simulink subsystem "rocket_flight"  (R2024b)
settings: Solver=VariableStepAuto  StartTime=0.0  StopTime=10.0  RelTol=1e-3
undefined symbols (not defined in the file or in its folder): location, Mdot, OR_cg, rail_angle_pitch, rail_angle_roll, rail_angle_yaw, sim_time, time_idle
libraries: shared6dof x1
settings Model: Creator=joedo  LastModifiedBy=finnb

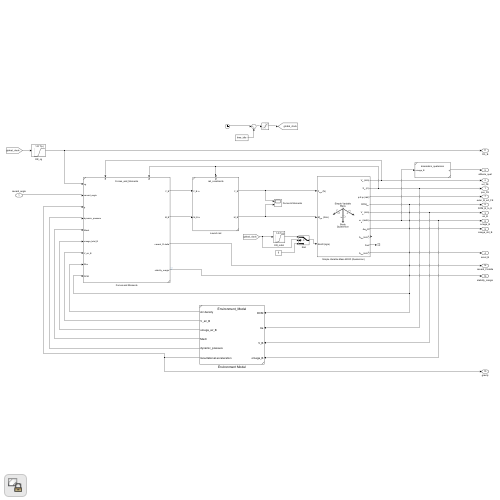
[thumbnail: Simulink's stored preview of the top-level diagram]
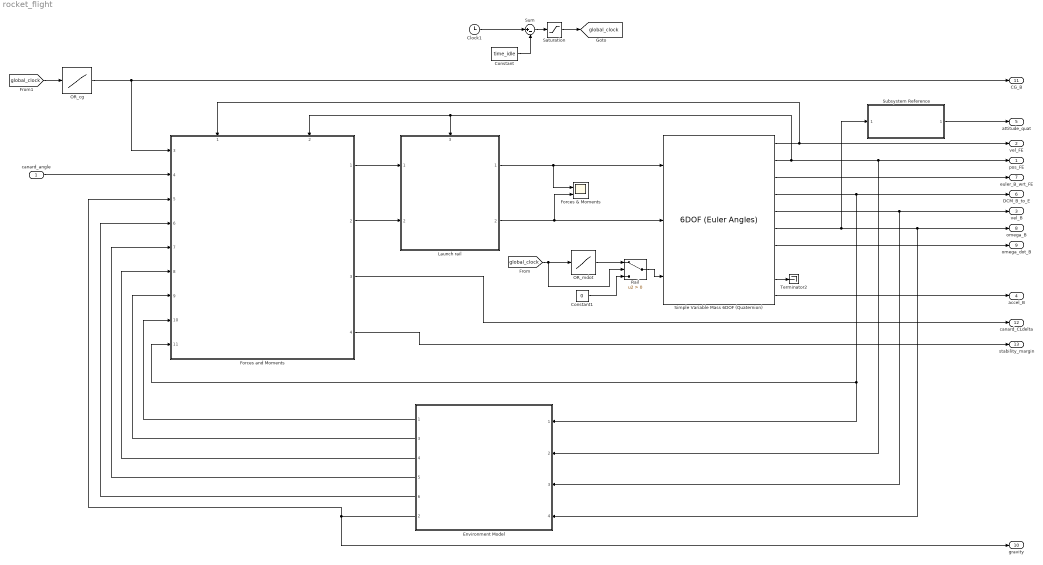
== system rocket_flight ==
  canard_angle : Inport
  Clock1 : Clock
  Constant : Constant  Value=time_idle
  Constant1 : Constant  Value=0
  Environment Model : Subsystem  ReferencedSubsystem=Environment_Model
      settings: PortSchema="{\"entries\":[{\"content\":{\"sides\":[{\"content\":{\"connectorIds\":[\"In1\",\"In2\",\"In3\",\"In4\"]},\"type\":\"ConnectorPlacement.EquallySpacedRectSide\",\"uuid\":\"2a81b9c5-b150-4b95-94af-394a03d0678a\"},{\"content\":{\"connectorIds\":[\"Out1\",\"Out3\",\"Out4\",\"Out5\",\"Out6\",\"Out2\"],\"side\":\"RIGHT\"},\"type\":\"ConnectorPlacement.EquallySpacedRectSide\",\"uuid\":\"876dc6e2-e5c6-4258-adc0-40f09f61a15a\"},{\"content\":{\"side\":\"TOP\"},\"type\":\"ConnectorPlacement.EquallySpacedRectSide\",\"uuid\":\"30ca8b3b-9b10-4b0a-a581-f2563a0e4844\"}]},\"type\":\"ConnectorPlacement.EquallySpacedConnector\",\"uuid\":\"0a44bd71-bf6b-4260-a474-a2581db635e7\"}],\"packageUris\":[\"http://schema.mathworks.com/mf0/Connector/R2020b\"],\"version\":\"1.0\"}"
  Forces & Moments : Scope  NumInputPorts=2
  "Forces and Moments " : Subsystem  ReferencedSubsystem=Forces_and_Moments
      settings: PortSchema="{\"entries\":[{\"content\":{\"sides\":[{\"content\":{\"connectorIds\":[\"In3\",\"In4\",\"In5\",\"In6\",\"In7\",\"In8\",\"In9\",\"In10\",\"In11\"]},\"type\":\"ConnectorPlacement.EquallySpacedRectSide\",\"uuid\":\"2d9b15f2-fc7e-4399-b4ca-f7faa58838df\"},{\"content\":{\"connectorIds\":[\"Out1\",\"Out2\",\"Out3\",\"Out4\"],\"side\":\"RIGHT\"},\"type\":\"ConnectorPlacement.EquallySpacedRectSide\",\"uuid\":\"cd9b89d4-ce85-488b-9a3f-64297ccf9b96\"},{\"content\":{\"connectorIds\":[\"In1\",\"In2\"],\"side\":\"TOP\"},\"type\":\"ConnectorPlacement.EquallySpacedRectSide\",\"uuid\":\"472a10a7-0072-45c6-a8aa-5eaf234894da\"}]},\"type\":\"ConnectorPlacement.EquallySpacedConnector\",\"uuid\":\"79d150c0-9861-42cf-8cdc-8f9e609deb28\"}],\"packageUris\":[\"http://schema.mathworks.com/mf0/Connector/R2020b\"],\"version\":\"1.0\"}"
  Launch rail : Subsystem  ReferencedSubsystem=rail_constraints
      settings: PortSchema="{\"entries\":[{\"content\":{\"sides\":[{\"content\":{\"connectorIds\":[\"In1\",\"In2\"]},\"type\":\"ConnectorPlacement.EquallySpacedRectSide\",\"uuid\":\"f8bc89cf-4366-4095-a699-e573bc22001a\"},{\"content\":{\"connectorIds\":[\"Out1\",\"Out2\"],\"side\":\"RIGHT\"},\"type\":\"ConnectorPlacement.EquallySpacedRectSide\",\"uuid\":\"f55d6fa0-3d5e-48fa-b07b-9e72276225fb\"},{\"content\":{\"connectorIds\":[\"In3\"],\"side\":\"TOP\"},\"type\":\"ConnectorPlacement.EquallySpacedRectSide\",\"uuid\":\"5696589c-23a4-46a9-b349-1864b914459a\"}]},\"type\":\"ConnectorPlacement.EquallySpacedConnector\",\"uuid\":\"1b8f695c-cf97-4880-abd1-8dadf97d6ecb\"}],\"packageUris\":[\"http://schema.mathworks.com/mf0/Connector/R2020b\"],\"version\":\"1.0\"}"
  OR_cg : Lookup_n-D  NumberOfTableDimensions=1  BreakpointsForDimension1=sim_time  Table=OR_cg  InternalRulePriority=Speed  RndMeth=Simplest
  OR_mdot : Lookup_n-D  NumberOfTableDimensions=1  BreakpointsForDimension1=sim_time  Table=Mdot  InternalRulePriority=Speed  RndMeth=Simplest
  Rail : Switch  Criteria=u2 > Threshold  SaturateOnIntegerOverflow=off  InputSameDT=off
  Saturation : Saturate  UpperLimit=inf  LowerLimit=0
  Simple Variable Mass 6DOF (Quaternion) : shared6dof/6DOF (Euler Angles)  units=Metric (MKS)  mtype=Simple Variable  rep=Quaternion  xme_0=[location(1) 0 0]  Vm_0=[0 0 0]  eul_0=[rail_angle_roll, rail_angle_pitch, rail_angle_yaw]  pm_0=[0 0 0]  mass_0=total_mass_0  mass_e=total_mass_d  mass_f=total_mass_0  inertia=eye(3)  inertia_e=I_d  inertia_f=I_0  k_quat=1.0  vre_flag=off  abi_flag=on  aMode=0  xme_statename=''  Vm_statename=''  eul_statename=''  quat_statename=''  pm_statename=''  mass_statename=''
      settings: LibrarySourceBlock=aerolib6dof2/Simple Variable Mass 6DOF (Quaternion)
  Subsystem Reference : Subsystem  ReferencedSubsystem=kinematics_quaternion
  Sum : Sum  Inputs=|+-
  Terminator2 : Terminator
  pos_FE : Outport
  vel_FE : Outport  Port=2
  vel_B : Outport  Port=3  PortDimensions=3
  accel_B : Outport  Port=4  PortDimensions=3
  attitude_quat : Outport  Port=5
  DCM_B_to_E : Outport  Port=6
  euler_B_wrt_FE : Outport  Port=7
  omega_B : Outport  Port=8
  omega_dot_B : Outport  Port=9
  gravity : Outport  Port=10
  CG_B : Outport  Port=11
  canard_CLdelta : Outport  Port=12
  stability_margin : Outport  Port=13
  tag scope: global_clock=global
  wires:
  "Forces and Moments "/4 -> stability_margin/1
  "Forces and Moments "/3 -> canard_CLdelta/1
  "Forces and Moments "/2 -> Launch rail/2
  "Forces and Moments "/1 -> Launch rail/1
  Environment Model/6 -> "Forces and Moments "/6
  Environment Model/3 -> "Forces and Moments "/9
  Subsystem Reference/1 -> attitude_quat/1
  Saturation/1 -> [global_clock]
  Constant/1 -> Sum/2
  Sum/1 -> Saturation/1
  Clock1/1 -> Sum/1
  OR_cg/1 -> "Forces and Moments "/3, CG_B/1
  [global_clock] -> OR_cg/1
  Constant1/1 -> Rail/3
  Rail/1 -> Simple Variable Mass 6DOF (Quaternion)/3
  [global_clock] -> OR_mdot/1, Rail/2
  Simple Variable Mass 6DOF (Quaternion)/4 -> Environment Model/1, "Forces and Moments "/11, DCM_B_to_E/1
  Simple Variable Mass 6DOF (Quaternion)/7 -> omega_dot_B/1
  Simple Variable Mass 6DOF (Quaternion)/3 -> euler_B_wrt_FE/1
  Simple Variable Mass 6DOF (Quaternion)/1 -> vel_FE/1, "Forces and Moments "/1
  Environment Model/2 -> gravity/1, "Forces and Moments "/5
  Simple Variable Mass 6DOF (Quaternion)/9 -> Terminator2/1
  Simple Variable Mass 6DOF (Quaternion)/10 -> accel_B/1
  OR_mdot/1 -> Rail/1
  Environment Model/5 -> "Forces and Moments "/7
  Simple Variable Mass 6DOF (Quaternion)/2 -> Environment Model/2, pos_FE/1, "Forces and Moments "/2, Launch rail/3
  Launch rail/2 -> Simple Variable Mass 6DOF (Quaternion)/2, Forces & Moments/2
  Environment Model/1 -> "Forces and Moments "/10
  Environment Model/4 -> "Forces and Moments "/8
  Simple Variable Mass 6DOF (Quaternion)/5 -> Environment Model/3, vel_B/1
  Simple Variable Mass 6DOF (Quaternion)/6 -> Subsystem Reference/1, Environment Model/4, omega_B/1
  canard_angle/1 -> "Forces and Moments "/4
  Launch rail/1 -> Forces & Moments/1, Simple Variable Mass 6DOF (Quaternion)/1
